simulink model "CF009A_GmOvrlStMgr"  (R2013b)
settings: Solver=FixedStepDiscrete  SolverMode=SingleTasking  StartTime=0.0  StopTime=1  FixedStep=0.002  RelTol=1e-3
values from neighbouring files (symbols this model uses):
  APASTACTV_CNT_U08 = DataDict.Constant    [CF009A_GmOvrlStMgr_DataDict.m]
  APASTCTRLAVL_CNT_U08 = DataDict.Constant    [CF009A_GmOvrlStMgr_DataDict.m]
  ARCHGLBPRM_2MILLISEC_SEC_F32 = DataDict.Constant    [CF009A_GmOvrlStMgr_DataDict.m]
  GmOvrlStMgrApaHwTqThd = DataDict.Calibration    [CF009A_GmOvrlStMgr_DataDict.m]
  GmOvrlStMgrApaHwTqTiThd = DataDict.Calibration    [CF009A_GmOvrlStMgr_DataDict.m]
  GmOvrlStMgrApaMfgEna = DataDict.Calibration    [CF009A_GmOvrlStMgr_DataDict.m]
  GmOvrlStMgrEscMfgEna = DataDict.Calibration    [CF009A_GmOvrlStMgr_DataDict.m]
  GmOvrlStMgrHaptcAmp = DataDict.Calibration    [CF009A_GmOvrlStMgr_DataDict.m]
  GmOvrlStMgrHaptcDurn = DataDict.Calibration    [CF009A_GmOvrlStMgr_DataDict.m]
  GmOvrlStMgrHaptcFrq = DataDict.Calibration    [CF009A_GmOvrlStMgr_DataDict.m]
  GmOvrlStMgrHaptcReactnTi = DataDict.Calibration    [CF009A_GmOvrlStMgr_DataDict.m]
  GmOvrlStMgrHaptcReqTiThd = DataDict.Calibration    [CF009A_GmOvrlStMgr_DataDict.m]
  GmOvrlStMgrHwAgTarLimr = DataDict.Calibration    [CF009A_GmOvrlStMgr_DataDict.m]
  GmOvrlStMgrLkaHwTqThd1 = DataDict.Calibration    [CF009A_GmOvrlStMgr_DataDict.m]
  GmOvrlStMgrLkaHwTqThd2 = DataDict.Calibration    [CF009A_GmOvrlStMgr_DataDict.m]
  GmOvrlStMgrLkaHwTqTiThd1 = DataDict.Calibration    [CF009A_GmOvrlStMgr_DataDict.m]
  GmOvrlStMgrLkaHwTqTiThd2 = DataDict.Calibration    [CF009A_GmOvrlStMgr_DataDict.m]
  GmOvrlStMgrLkaMfgEna = DataDict.Calibration    [CF009A_GmOvrlStMgr_DataDict.m]
  GmOvrlStMgrLoaMtgtnHaptcFbOffTi = DataDict.Calibration    [CF009A_GmOvrlStMgr_DataDict.m]
  GmOvrlStMgrLoaMtgtnHaptcFbOnTi = DataDict.Calibration    [CF009A_GmOvrlStMgr_DataDict.m]
  GmOvrlStMgrLoaMtgtnHaptcFbStrtOnTi = DataDict.Calibration    [CF009A_GmOvrlStMgr_DataDict.m]
  GmOvrlStMgrLoaMtgtnHaptcFbTqMax = DataDict.Calibration    [CF009A_GmOvrlStMgr_DataDict.m]
  GmOvrlStMgrLoaMtgtnHaptcFbTqMin = DataDict.Calibration    [CF009A_GmOvrlStMgr_DataDict.m]
  GmOvrlStMgrLoaMtgtnHaptcFbVehSpdMax = DataDict.Calibration    [CF009A_GmOvrlStMgr_DataDict.m]
  GmOvrlStMgrLoaMtgtnHaptcFbVehSpdMin = DataDict.Calibration    [CF009A_GmOvrlStMgr_DataDict.m]
  GmOvrlStMgrLoaMtgtnHaptcFrq = DataDict.Calibration    [CF009A_GmOvrlStMgr_DataDict.m]
  GmOvrlStMgrLoaMtgtnStrtHaptcAmp = DataDict.Calibration    [CF009A_GmOvrlStMgr_DataDict.m]
  GmOvrlStMgrLoaStIgnCntrThd = DataDict.Calibration    [CF009A_GmOvrlStMgr_DataDict.m]
  GmOvrlStMgrShiftLvrTiThd = DataDict.Calibration    [CF009A_GmOvrlStMgr_DataDict.m]
  GmOvrlStMgrStandStillThd = DataDict.Calibration    [CF009A_GmOvrlStMgr_DataDict.m]
  GmOvrlStMgrStandStillTiThd = DataDict.Calibration    [CF009A_GmOvrlStMgr_DataDict.m]
  HAPTCSTACTV_CNT_U08 = DataDict.Constant    [CF009A_GmOvrlStMgr_DataDict.m]
  HAPTCSTWAIT_CNT_U08 = DataDict.Constant    [CF009A_GmOvrlStMgr_DataDict.m]
  HWOSCNFRQMIN_HZ_F32 = DataDict.Constant    [CF009A_GmOvrlStMgr_DataDict.m]
  LKAFLTCNTRTHD_CNT_U08 = DataDict.Constant    [CF009A_GmOvrlStMgr_DataDict.m]
  LKAFLTTMRTHD_MILLISEC_U32 = DataDict.Constant    [CF009A_GmOvrlStMgr_DataDict.m]
  LKASTPRMNTFAILD_CNT_U08 = DataDict.Constant    [CF009A_GmOvrlStMgr_DataDict.m]
  LoaMtgtnThdExcdd = DataDict.NTC    [CF009A_GmOvrlStMgr_DataDict.m]
  MILLISECTO100MICROSECCNVN_CNT_U32 = DataDict.Constant    [CF009A_GmOvrlStMgr_DataDict.m]
  NODEBSTEP_CNT_U16 = DataDict.Constant    [CF009A_GmOvrlStMgr_DataDict.m]
undefined symbols (not defined in the file or in its folder): LoaSt1, NtcSts1, NVM_RequestResultType, SysSt1
libraries: simulink x13, Fil x6, NxtrNvM x4, NxtrLim x4, NxtrAbslt x3, NxtrSign x2, FixdToFloat x1, FloatToFixd x1, LnrIntrpn x1
(part 6 of 8)

== system CF009A_GmOvrlStMgr/GmOvrlStMgr/GmOvrlStMgrPer1/Timer for HwHaptcEna/If Action Subsystem/GetRefTmr100MicroSec32bit ==
  note: GetRefTmr100MicroSec32bit
  note: Wrap-to-zero
  note: counts
  note: microseconds
  note: seconds
  note: 1 count = 100 uSec
  CopyRight2 : Subsystem  Description=|  mask(Copyright Information){none=on}
      | Copyright info block.                                               
      |                                                                     
      | Place copyright information at the top of every subsystem in design.
      mask prompts: none "No parameters"
      mask help: Place copyright information at the top of every subsystem in design.
      mask Display:
      | NxtrConf = 'Nexteer Confidential';
      | 
      | sys = bdroot; %handle for the current model ("system")
      | first = get_param(sys,'Created');
      | if(isempty(first))
      |     first = datestr(now,'yyyy');
      | else
      |     first = first(end-3:end);  %year is last four digits
      | end
      | 
      | last = get_param(sys,'LastModifiedDate');
      | if isempty(last)
      |     last = datestr(now,'yyyy');
      | else
      |     last = last(end-3:end);
      | end
      | 
      | if strcmp(first,last)
      |     fprintf('%s -- Copyright %s Nexteer',NxtrConf,first)
      | else
      |     fprintf('%s -- %s%s- %s Nexteer',NxtrConf,char(169),first,last)
      | end
  Count per uSec : Constant  Value=0.01
  Data Store Read1 : DataStoreRead  DataStoreName=SimnTi
  Data Type Conversion1 : DataTypeConversion  OutDataTypeStr=uint32
  Divide1 : Product  Inputs=**
  Divide2 : Product  Inputs=*/
  Max Counts : Constant  Value=2^32-1
  Product1 : Product
  Product2 : Product
  Rounding : Rounding
  Subtract1 : Sum  Inputs=+-
  uSec per Sec : Constant  Value=1000000
  RefTmr : Outport
  wires:
  Data Type Conversion1/1 -> RefTmr/1
  uSec per Sec/1 -> Product1/2
  Count per uSec/1 -> Divide1/2
  Data Store Read1/1 -> Product1/1
  Product1/1 -> Divide1/1
  Divide1/1 -> Subtract1/1, Divide2/1
  Max Counts/1 -> Product2/2, Divide2/2
  Divide2/1 -> Rounding/1
  Rounding/1 -> Product2/1
  Subtract1/1 -> Data Type Conversion1/1
  Product2/1 -> Subtract1/2

== system CF009A_GmOvrlStMgr/GmOvrlStMgr/GmOvrlStMgrPer1/Timer for HwHaptcEna/If Action Subsystem1/CopyRight2 ==

== system CF009A_GmOvrlStMgr/GmOvrlStMgr/GmOvrlStMgrPer1/Timer for HwHaptcEna/If Action Subsystem2/CopyRight2 ==

== system CF009A_GmOvrlStMgr/GmOvrlStMgr/GmOvrlStMgrPer1/Timer for HwHaptcEna/If Action Subsystem2/GetTiSpan100MicroSec32bit1 ==
  note: GetTiSpan100MicroSec32bit
  note: Get current system time
  note: 1 count = 100 uSec
  note: Wrap-to-zero
  note: counts
  note: microseconds
  note: seconds
  note: Subtract original reference time
  RefTmr : Inport
  CopyRight2 : Subsystem  Description=|  mask(Copyright Information){none=on}
      | Copyright info block.                                               
      |                                                                     
      | Place copyright information at the top of every subsystem in design.
      mask prompts: none "No parameters"
      mask help: Place copyright information at the top of every subsystem in design.
      mask Display:
      | NxtrConf = 'Nexteer Confidential';
      | 
      | sys = bdroot; %handle for the current model ("system")
      | first = get_param(sys,'Created');
      | if(isempty(first))
      |     first = datestr(now,'yyyy');
      | else
      |     first = first(end-3:end);  %year is last four digits
      | end
      | 
      | last = get_param(sys,'LastModifiedDate');
      | if isempty(last)
      |     last = datestr(now,'yyyy');
      | else
      |     last = last(end-3:end);
      | end
      | 
      | if strcmp(first,last)
      |     fprintf('%s -- Copyright %s Nexteer',NxtrConf,first)
      | else
      |     fprintf('%s -- %s%s- %s Nexteer',NxtrConf,char(169),first,last)
      | end
  Count per uSec : Constant  Value=0.01
  Data Store Read1 : DataStoreRead  DataStoreName=SimnTi
  Data Type Conversion2 : DataTypeConversion  OutDataTypeStr=uint32
  Divide1 : Product  Inputs=**
  Divide2 : Product  Inputs=*/
  If : If  NumInputs=2  IfExpression=u1 >= u2
  Max Counts : Constant  Value=2^32-1
  Merge : Merge
  No wrapping : Subsystem  TreatAsAtomicUnit=on
  Product2 : Product
  Product3 : Product
  Rounding : Rounding
  Subtract3 : Sum  Inputs=+-
  Wrapping : Subsystem  TreatAsAtomicUnit=on
  uSec per Sec : Constant  Value=1000000
  TiSpan : Outport
  wires:
  Data Type Conversion2/1 -> Wrapping/1(new), No wrapping/1(new), If/1
  RefTmr/1 -> Wrapping/2(ref), No wrapping/2(ref), If/2
  Merge/1 -> TiSpan/1
  uSec per Sec/1 -> Product2/2
  Count per uSec/1 -> Divide1/2
  Data Store Read1/1 -> Product2/1
  Product2/1 -> Divide1/1
  Divide1/1 -> Subtract3/1, Divide2/1
  Max Counts/1 -> Product3/2, Divide2/2
  Divide2/1 -> Rounding/1
  Rounding/1 -> Product3/1
  Subtract3/1 -> Data Type Conversion2/1
  Product3/1 -> Subtract3/2
  If/1 -> No wrapping/Action
  If/2 -> Wrapping/Action
  No wrapping/1(Out1) -> Merge/1
  Wrapping/1(Out1) -> Merge/2

== system CF009A_GmOvrlStMgr/GmOvrlStMgr/GmOvrlStMgrPer1/Timer for ShiftLvrRvs/If Action Subsystem/CopyRight2 ==

== system CF009A_GmOvrlStMgr/GmOvrlStMgr/GmOvrlStMgrPer1/Timer for ShiftLvrRvs/If Action Subsystem/GetRefTmr100MicroSec32bit ==
  note: GetRefTmr100MicroSec32bit
  note: Wrap-to-zero
  note: counts
  note: microseconds
  note: seconds
  note: 1 count = 100 uSec
  CopyRight2 : Subsystem  Description=|  mask(Copyright Information){none=on}
      | Copyright info block.                                               
      |                                                                     
      | Place copyright information at the top of every subsystem in design.
      mask prompts: none "No parameters"
      mask help: Place copyright information at the top of every subsystem in design.
      mask Display:
      | NxtrConf = 'Nexteer Confidential';
      | 
      | sys = bdroot; %handle for the current model ("system")
      | first = get_param(sys,'Created');
      | if(isempty(first))
      |     first = datestr(now,'yyyy');
      | else
      |     first = first(end-3:end);  %year is last four digits
      | end
      | 
      | last = get_param(sys,'LastModifiedDate');
      | if isempty(last)
      |     last = datestr(now,'yyyy');
      | else
      |     last = last(end-3:end);
      | end
      | 
      | if strcmp(first,last)
      |     fprintf('%s -- Copyright %s Nexteer',NxtrConf,first)
      | else
      |     fprintf('%s -- %s%s- %s Nexteer',NxtrConf,char(169),first,last)
      | end
  Count per uSec : Constant  Value=0.01
  Data Store Read1 : DataStoreRead  DataStoreName=SimnTi
  Data Type Conversion1 : DataTypeConversion  OutDataTypeStr=uint32
  Divide1 : Product  Inputs=**
  Divide2 : Product  Inputs=*/
  Max Counts : Constant  Value=2^32-1
  Product1 : Product
  Product2 : Product
  Rounding : Rounding
  Subtract1 : Sum  Inputs=+-
  uSec per Sec : Constant  Value=1000000
  RefTmr : Outport
  wires:
  Data Type Conversion1/1 -> RefTmr/1
  uSec per Sec/1 -> Product1/2
  Count per uSec/1 -> Divide1/2
  Data Store Read1/1 -> Product1/1
  Product1/1 -> Divide1/1
  Divide1/1 -> Subtract1/1, Divide2/1
  Max Counts/1 -> Product2/2, Divide2/2
  Divide2/1 -> Rounding/1
  Rounding/1 -> Product2/1
  Subtract1/1 -> Data Type Conversion1/1
  Product2/1 -> Subtract1/2

== system CF009A_GmOvrlStMgr/GmOvrlStMgr/GmOvrlStMgrPer1/Timer for ShiftLvrRvs/If Action Subsystem1/CopyRight2 ==

== system CF009A_GmOvrlStMgr/GmOvrlStMgr/GmOvrlStMgrPer1/Timer for ShiftLvrRvs/If Action Subsystem2/CopyRight2 ==

== system CF009A_GmOvrlStMgr/GmOvrlStMgr/GmOvrlStMgrPer1/Timer for ShiftLvrRvs/If Action Subsystem2/GetTiSpan100MicroSec32bit1 ==
  note: GetTiSpan100MicroSec32bit
  note: Get current system time
  note: 1 count = 100 uSec
  note: Wrap-to-zero
  note: counts
  note: microseconds
  note: seconds
  note: Subtract original reference time
  RefTmr : Inport
  CopyRight2 : Subsystem  Description=|  mask(Copyright Information){none=on}
      | Copyright info block.                                               
      |                                                                     
      | Place copyright information at the top of every subsystem in design.
      mask prompts: none "No parameters"
      mask help: Place copyright information at the top of every subsystem in design.
      mask Display:
      | NxtrConf = 'Nexteer Confidential';
      | 
      | sys = bdroot; %handle for the current model ("system")
      | first = get_param(sys,'Created');
      | if(isempty(first))
      |     first = datestr(now,'yyyy');
      | else
      |     first = first(end-3:end);  %year is last four digits
      | end
      | 
      | last = get_param(sys,'LastModifiedDate');
      | if isempty(last)
      |     last = datestr(now,'yyyy');
      | else
      |     last = last(end-3:end);
      | end
      | 
      | if strcmp(first,last)
      |     fprintf('%s -- Copyright %s Nexteer',NxtrConf,first)
      | else
      |     fprintf('%s -- %s%s- %s Nexteer',NxtrConf,char(169),first,last)
      | end
  Count per uSec : Constant  Value=0.01
  Data Store Read1 : DataStoreRead  DataStoreName=SimnTi
  Data Type Conversion2 : DataTypeConversion  OutDataTypeStr=uint32
  Divide1 : Product  Inputs=**
  Divide2 : Product  Inputs=*/
  If : If  NumInputs=2  IfExpression=u1 >= u2
  Max Counts : Constant  Value=2^32-1
  Merge : Merge
  No wrapping : Subsystem  TreatAsAtomicUnit=on
  Product2 : Product
  Product3 : Product
  Rounding : Rounding
  Subtract3 : Sum  Inputs=+-
  Wrapping : Subsystem  TreatAsAtomicUnit=on
  uSec per Sec : Constant  Value=1000000
  TiSpan : Outport
  wires:
  Data Type Conversion2/1 -> Wrapping/1(new), No wrapping/1(new), If/1
  RefTmr/1 -> Wrapping/2(ref), No wrapping/2(ref), If/2
  Merge/1 -> TiSpan/1
  uSec per Sec/1 -> Product2/2
  Count per uSec/1 -> Divide1/2
  Data Store Read1/1 -> Product2/1
  Product2/1 -> Divide1/1
  Divide1/1 -> Subtract3/1, Divide2/1
  Max Counts/1 -> Product3/2, Divide2/2
  Divide2/1 -> Rounding/1
  Rounding/1 -> Product3/1
  Subtract3/1 -> Data Type Conversion2/1
  Product3/1 -> Subtract3/2
  If/1 -> No wrapping/Action
  If/2 -> Wrapping/Action
  No wrapping/1(Out1) -> Merge/1
  Wrapping/1(Out1) -> Merge/2

== system CF009A_GmOvrlStMgr/GmOvrlStMgr/GmOvrlStMgrPer1/Timer for VehStandStill/If Action Subsystem/CopyRight2 ==

== system CF009A_GmOvrlStMgr/GmOvrlStMgr/GmOvrlStMgrPer1/Timer for VehStandStill/If Action Subsystem/GetRefTmr100MicroSec32bit ==
  note: GetRefTmr100MicroSec32bit
  note: Wrap-to-zero
  note: counts
  note: microseconds
  note: seconds
  note: 1 count = 100 uSec
  CopyRight2 : Subsystem  Description=|  mask(Copyright Information){none=on}
      | Copyright info block.                                               
      |                                                                     
      | Place copyright information at the top of every subsystem in design.
      mask prompts: none "No parameters"
      mask help: Place copyright information at the top of every subsystem in design.
      mask Display:
      | NxtrConf = 'Nexteer Confidential';
      | 
      | sys = bdroot; %handle for the current model ("system")
      | first = get_param(sys,'Created');
      | if(isempty(first))
      |     first = datestr(now,'yyyy');
      | else
      |     first = first(end-3:end);  %year is last four digits
      | end
      | 
      | last = get_param(sys,'LastModifiedDate');
      | if isempty(last)
      |     last = datestr(now,'yyyy');
      | else
      |     last = last(end-3:end);
      | end
      | 
      | if strcmp(first,last)
      |     fprintf('%s -- Copyright %s Nexteer',NxtrConf,first)
      | else
      |     fprintf('%s -- %s%s- %s Nexteer',NxtrConf,char(169),first,last)
      | end
  Count per uSec : Constant  Value=0.01
  Data Store Read1 : DataStoreRead  DataStoreName=SimnTi
  Data Type Conversion1 : DataTypeConversion  OutDataTypeStr=uint32
  Divide1 : Product  Inputs=**
  Divide2 : Product  Inputs=*/
  Max Counts : Constant  Value=2^32-1
  Product1 : Product
  Product2 : Product
  Rounding : Rounding
  Subtract1 : Sum  Inputs=+-
  uSec per Sec : Constant  Value=1000000
  RefTmr : Outport
  wires:
  Data Type Conversion1/1 -> RefTmr/1
  uSec per Sec/1 -> Product1/2
  Count per uSec/1 -> Divide1/2
  Data Store Read1/1 -> Product1/1
  Product1/1 -> Divide1/1
  Divide1/1 -> Subtract1/1, Divide2/1
  Max Counts/1 -> Product2/2, Divide2/2
  Divide2/1 -> Rounding/1
  Rounding/1 -> Product2/1
  Subtract1/1 -> Data Type Conversion1/1
  Product2/1 -> Subtract1/2

== system CF009A_GmOvrlStMgr/GmOvrlStMgr/GmOvrlStMgrPer1/Timer for VehStandStill/If Action Subsystem1/CopyRight2 ==

== system CF009A_GmOvrlStMgr/GmOvrlStMgr/GmOvrlStMgrPer1/Timer for VehStandStill/If Action Subsystem2/CopyRight2 ==

== system CF009A_GmOvrlStMgr/GmOvrlStMgr/GmOvrlStMgrPer1/Timer for VehStandStill/If Action Subsystem2/GetTiSpan100MicroSec32bit1 ==
  note: GetTiSpan100MicroSec32bit
  note: Get current system time
  note: 1 count = 100 uSec
  note: Wrap-to-zero
  note: counts
  note: microseconds
  note: seconds
  note: Subtract original reference time
  RefTmr : Inport
  CopyRight2 : Subsystem  Description=|  mask(Copyright Information){none=on}
      | Copyright info block.                                               
      |                                                                     
      | Place copyright information at the top of every subsystem in design.
      mask prompts: none "No parameters"
      mask help: Place copyright information at the top of every subsystem in design.
      mask Display:
      | NxtrConf = 'Nexteer Confidential';
      | 
      | sys = bdroot; %handle for the current model ("system")
      | first = get_param(sys,'Created');
      | if(isempty(first))
      |     first = datestr(now,'yyyy');
      | else
      |     first = first(end-3:end);  %year is last four digits
      | end
      | 
      | last = get_param(sys,'LastModifiedDate');
      | if isempty(last)
      |     last = datestr(now,'yyyy');
      | else
      |     last = last(end-3:end);
      | end
      | 
      | if strcmp(first,last)
      |     fprintf('%s -- Copyright %s Nexteer',NxtrConf,first)
      | else
      |     fprintf('%s -- %s%s- %s Nexteer',NxtrConf,char(169),first,last)
      | end
  Count per uSec : Constant  Value=0.01
  Data Store Read1 : DataStoreRead  DataStoreName=SimnTi
  Data Type Conversion2 : DataTypeConversion  OutDataTypeStr=uint32
  Divide1 : Product  Inputs=**
  Divide2 : Product  Inputs=*/
  If : If  NumInputs=2  IfExpression=u1 >= u2
  Max Counts : Constant  Value=2^32-1
  Merge : Merge
  No wrapping : Subsystem  TreatAsAtomicUnit=on
  Product2 : Product
  Product3 : Product
  Rounding : Rounding
  Subtract3 : Sum  Inputs=+-
  Wrapping : Subsystem  TreatAsAtomicUnit=on
  uSec per Sec : Constant  Value=1000000
  TiSpan : Outport
  wires:
  Data Type Conversion2/1 -> Wrapping/1(new), No wrapping/1(new), If/1
  RefTmr/1 -> Wrapping/2(ref), No wrapping/2(ref), If/2
  Merge/1 -> TiSpan/1
  uSec per Sec/1 -> Product2/2
  Count per uSec/1 -> Divide1/2
  Data Store Read1/1 -> Product2/1
  Product2/1 -> Divide1/1
  Divide1/1 -> Subtract3/1, Divide2/1
  Max Counts/1 -> Product3/2, Divide2/2
  Divide2/1 -> Rounding/1
  Rounding/1 -> Product3/1
  Subtract3/1 -> Data Type Conversion2/1
  Product3/1 -> Subtract3/2
  If/1 -> No wrapping/Action
  If/2 -> Wrapping/Action
  No wrapping/1(Out1) -> Merge/1
  Wrapping/1(Out1) -> Merge/2

== system CF009A_GmOvrlStMgr/GmOvrlStMgr/GmOvrlStMgrPer1/TransHaptcsWaitToAPAStActvFlg/ElpseTi/CopyRight2 ==

== system CF009A_GmOvrlStMgr/GmOvrlStMgr/GmOvrlStMgrPer1/TransHaptcsWaitToAPAStActvFlg/ElpseTi/GetTiSpan100MicroSec32bit ==
  note: Created Aug 18, 2015
      | Modified Oct 21, 2015
      | Modified Oct 30, 2015
      | Kevin Derry
  note: GetTiSpan100MicroSec32bit
  note: Get current system time
  note: 1 count = 100 uSec
  note: Wrap-to-zero
  note: counts
  note: microseconds
  note: seconds
  note: Subtract original reference time
  RefTmr : Inport
  CopyRight2 : Subsystem  Description=|  mask(Copyright Information){none=on}
      | Copyright info block.                                               
      |                                                                     
      | Place copyright information at the top of every subsystem in design.
      mask prompts: none "No parameters"
      mask help: Place copyright information at the top of every subsystem in design.
      mask Display:
      | NxtrConf = 'Nexteer Confidential';
      | 
      | sys = bdroot; %handle for the current model ("system")
      | first = get_param(sys,'Created');
      | if(isempty(first))
      |     first = datestr(now,'yyyy');
      | else
      |     first = first(end-3:end);  %year is last four digits
      | end
      | 
      | last = get_param(sys,'LastModifiedDate');
      | if isempty(last)
      |     last = datestr(now,'yyyy');
      | else
      |     last = last(end-3:end);
      | end
      | 
      | if strcmp(first,last)
      |     fprintf('%s -- Copyright %s Nexteer',NxtrConf,first)
      | else
      |     fprintf('%s -- %s%s- %s Nexteer',NxtrConf,char(169),first,last)
      | end
  Count per uSec : Constant  Value=0.01
  Data Store Read1 : DataStoreRead  DataStoreName=SimnTi
  Data Type Conversion2 : DataTypeConversion  OutDataTypeStr=uint32
  Divide1 : Product  Inputs=**
  Divide2 : Product  Inputs=*/
  If : If  NumInputs=2  IfExpression=u1 >= u2
  Max Counts : Constant  Value=2^32-1
  Merge : Merge
  No wrapping : Subsystem  TreatAsAtomicUnit=on
  Product2 : Product
  Product3 : Product
  Rounding : Rounding
  Subtract3 : Sum  Inputs=+-
  Wrapping : Subsystem  TreatAsAtomicUnit=on
  uSec per Sec : Constant  Value=1000000
  TiSpan : Outport
  wires:
  Data Type Conversion2/1 -> Wrapping/1(new), No wrapping/1(new), If/1
  RefTmr/1 -> Wrapping/2(ref), No wrapping/2(ref), If/2
  Merge/1 -> TiSpan/1
  uSec per Sec/1 -> Product2/2
  Count per uSec/1 -> Divide1/2
  Data Store Read1/1 -> Product2/1
  Product2/1 -> Divide1/1
  Divide1/1 -> Subtract3/1, Divide2/1
  Max Counts/1 -> Product3/2, Divide2/2
  Divide2/1 -> Rounding/1
  Rounding/1 -> Product3/1
  Subtract3/1 -> Data Type Conversion2/1
  Product3/1 -> Subtract3/2
  If/1 -> No wrapping/Action
  If/2 -> Wrapping/Action
  No wrapping/1(Out1) -> Merge/1
  Wrapping/1(Out1) -> Merge/2

== system CF009A_GmOvrlStMgr/GmOvrlStMgr/GmOvrlStMgrPer1/TransHaptcsWaitToAPAStActvFlg/ElpseTi/Set False Subsystem ==
  Action Port : ActionPort  ActionType=else
  Constant1 : Constant  RequirementInfo={} %GIDa_654f473a_f2a5_43e8_8504_41bd23fb1d71  Value=false  OutDataTypeStr=boolean
      settings: AttributesFormatString=%<OutDataTypeStr>
  CopyRight2 : Subsystem  Description=|  mask(Copyright Information){none=on}
      | Copyright info block.                                               
      |                                                                     
      | Place copyright information at the top of every subsystem in design.
      mask prompts: none "No parameters"
      mask help: Place copyright information at the top of every subsystem in design.
      mask Display:
      | NxtrConf = 'Nexteer Confidential';
      | 
      | sys = bdroot; %handle for the current model ("system")
      | first = get_param(sys,'Created');
      | first = first(end-3:end);  %year is last four digits
      | 
      | last = get_param(sys,'LastModifiedDate');
      | if isempty(last)
      |     last = datestr(now,'yyyy');
      | else
      |     last = last(end-3:end);
      | end
      | 
      | if strcmp(first,last)
      |     fprintf('%s -- Copyright %s Nexteer',NxtrConf,first)
      | else
      |     fprintf('%s -- %s%s- %s Nexteer',NxtrConf,char(169),first,last)
      | end
  Out1 : Outport
  wires:
  Constant1/1 -> Out1/1

== system CF009A_GmOvrlStMgr/GmOvrlStMgr/GmOvrlStMgrPer1/TransHaptcsWaitToAPAStActvFlg/ElpseTi/Set True Subsystem ==
  Action Port : ActionPort  ActionType=then
  Constant13 : Constant  RequirementInfo={} %GIDa_d24888ab_9be7_4cc6_a531_95638502a8a2  Value=true  OutDataTypeStr=boolean
      settings: AttributesFormatString=%<OutDataTypeStr>
  CopyRight2 : Subsystem  Description=|  mask(Copyright Information){none=on}
      | Copyright info block.                                               
      |                                                                     
      | Place copyright information at the top of every subsystem in design.
      mask prompts: none "No parameters"
      mask help: Place copyright information at the top of every subsystem in design.
      mask Display:
      | NxtrConf = 'Nexteer Confidential';
      | 
      | sys = bdroot; %handle for the current model ("system")
      | first = get_param(sys,'Created');
      | first = first(end-3:end);  %year is last four digits
      | 
      | last = get_param(sys,'LastModifiedDate');
      | if isempty(last)
      |     last = datestr(now,'yyyy');
      | else
      |     last = last(end-3:end);
      | end
      | 
      | if strcmp(first,last)
      |     fprintf('%s -- Copyright %s Nexteer',NxtrConf,first)
      | else
      |     fprintf('%s -- %s%s- %s Nexteer',NxtrConf,char(169),first,last)
      | end
  Out1 : Outport
  wires:
  Constant13/1 -> Out1/1

== system CF009A_GmOvrlStMgr/GmOvrlStMgr/GmOvrlStMgrPer1/TransHaptcsWaitToAPAStActvFlg/RefTi/CopyRight2 ==

== system CF009A_GmOvrlStMgr/GmOvrlStMgr/GmOvrlStMgrPer1/TransHaptcsWaitToAPAStActvFlg/RefTi/GetRefTmr100MicroSec32bit ==
  note: Created Aug 18, 2015
      | Modified Oct 21, 2015
      | Modified Oct 30, 2015
      | Kevin Derry
  note: GetRefTmr100MicroSec32bit
  note: Wrap-to-zero
  note: counts
  note: microseconds
  note: seconds
  note: 1 count = 100 uSec
  CopyRight2 : Subsystem  Description=|  mask(Copyright Information){none=on}
      | Copyright info block.                                               
      |                                                                     
      | Place copyright information at the top of every subsystem in design.
      mask prompts: none "No parameters"
      mask help: Place copyright information at the top of every subsystem in design.
      mask Display:
      | NxtrConf = 'Nexteer Confidential';
      | 
      | sys = bdroot; %handle for the current model ("system")
      | first = get_param(sys,'Created');
      | if(isempty(first))
      |     first = datestr(now,'yyyy');
      | else
      |     first = first(end-3:end);  %year is last four digits
      | end
      | 
      | last = get_param(sys,'LastModifiedDate');
      | if isempty(last)
      |     last = datestr(now,'yyyy');
      | else
      |     last = last(end-3:end);
      | end
      | 
      | if strcmp(first,last)
      |     fprintf('%s -- Copyright %s Nexteer',NxtrConf,first)
      | else
      |     fprintf('%s -- %s%s- %s Nexteer',NxtrConf,char(169),first,last)
      | end
  Count per uSec : Constant  Value=0.01
  Data Store Read1 : DataStoreRead  DataStoreName=SimnTi
  Data Type Conversion1 : DataTypeConversion  OutDataTypeStr=uint32
  Divide1 : Product  Inputs=**
  Divide2 : Product  Inputs=*/
  Max Counts : Constant  Value=2^32-1
  Product1 : Product
  Product2 : Product
  Rounding : Rounding
  Subtract1 : Sum  Inputs=+-
  uSec per Sec : Constant  Value=1000000
  RefTmr : Outport
  wires:
  Data Store Read1/1 -> Product1/1
  Data Type Conversion1/1 -> RefTmr/1
  uSec per Sec/1 -> Product1/2
  Count per uSec/1 -> Divide1/2
  Product1/1 -> Divide1/1
  Divide1/1 -> Subtract1/1, Divide2/1
  Max Counts/1 -> Product2/2, Divide2/2
  Divide2/1 -> Rounding/1
  Rounding/1 -> Product2/1
  Subtract1/1 -> Data Type Conversion1/1
  Product2/1 -> Subtract1/2

== system CF009A_GmOvrlStMgr/GmOvrlStMgr/GmOvrlStMgrPer1/ApaIntv/Timer for ApaIntv/If Action Subsystem/CopyRight2 ==

== system CF009A_GmOvrlStMgr/GmOvrlStMgr/GmOvrlStMgrPer1/ApaIntv/Timer for ApaIntv/If Action Subsystem/GetRefTmr100MicroSec32bit ==
  note: GetRefTmr100MicroSec32bit
  note: Wrap-to-zero
  note: counts
  note: microseconds
  note: seconds
  note: 1 count = 100 uSec
  CopyRight2 : Subsystem  Description=|  mask(Copyright Information){none=on}
      | Copyright info block.                                               
      |                                                                     
      | Place copyright information at the top of every subsystem in design.
      mask prompts: none "No parameters"
      mask help: Place copyright information at the top of every subsystem in design.
      mask Display:
      | NxtrConf = 'Nexteer Confidential';
      | 
      | sys = bdroot; %handle for the current model ("system")
      | first = get_param(sys,'Created');
      | if(isempty(first))
      |     first = datestr(now,'yyyy');
      | else
      |     first = first(end-3:end);  %year is last four digits
      | end
      | 
      | last = get_param(sys,'LastModifiedDate');
      | if isempty(last)
      |     last = datestr(now,'yyyy');
      | else
      |     last = last(end-3:end);
      | end
      | 
      | if strcmp(first,last)
      |     fprintf('%s -- Copyright %s Nexteer',NxtrConf,first)
      | else
      |     fprintf('%s -- %s%s- %s Nexteer',NxtrConf,char(169),first,last)
      | end
  Count per uSec : Constant  Value=0.01
  Data Store Read1 : DataStoreRead  DataStoreName=SimnTi
  Data Type Conversion1 : DataTypeConversion  OutDataTypeStr=uint32
  Divide1 : Product  Inputs=**
  Divide2 : Product  Inputs=*/
  Max Counts : Constant  Value=2^32-1
  Product1 : Product
  Product2 : Product
  Rounding : Rounding
  Subtract1 : Sum  Inputs=+-
  uSec per Sec : Constant  Value=1000000
  RefTmr : Outport
  wires:
  Data Type Conversion1/1 -> RefTmr/1
  uSec per Sec/1 -> Product1/2
  Count per uSec/1 -> Divide1/2
  Data Store Read1/1 -> Product1/1
  Product1/1 -> Divide1/1
  Divide1/1 -> Subtract1/1, Divide2/1
  Max Counts/1 -> Product2/2, Divide2/2
  Divide2/1 -> Rounding/1
  Rounding/1 -> Product2/1
  Subtract1/1 -> Data Type Conversion1/1
  Product2/1 -> Subtract1/2

== system CF009A_GmOvrlStMgr/GmOvrlStMgr/GmOvrlStMgrPer1/ApaIntv/Timer for ApaIntv/If Action Subsystem1/CopyRight2 ==

== system CF009A_GmOvrlStMgr/GmOvrlStMgr/GmOvrlStMgrPer1/ApaIntv/Timer for ApaIntv/If Action Subsystem2/CopyRight2 ==

== system CF009A_GmOvrlStMgr/GmOvrlStMgr/GmOvrlStMgrPer1/ApaIntv/Timer for ApaIntv/If Action Subsystem2/GetTiSpan100MicroSec32bit1 ==
  note: GetTiSpan100MicroSec32bit
  note: Get current system time
  note: 1 count = 100 uSec
  note: Wrap-to-zero
  note: counts
  note: microseconds
  note: seconds
  note: Subtract original reference time
  RefTmr : Inport
  CopyRight2 : Subsystem  Description=|  mask(Copyright Information){none=on}
      | Copyright info block.                                               
      |                                                                     
      | Place copyright information at the top of every subsystem in design.
      mask prompts: none "No parameters"
      mask help: Place copyright information at the top of every subsystem in design.
      mask Display:
      | NxtrConf = 'Nexteer Confidential';
      | 
      | sys = bdroot; %handle for the current model ("system")
      | first = get_param(sys,'Created');
      | if(isempty(first))
      |     first = datestr(now,'yyyy');
      | else
      |     first = first(end-3:end);  %year is last four digits
      | end
      | 
      | last = get_param(sys,'LastModifiedDate');
      | if isempty(last)
      |     last = datestr(now,'yyyy');
      | else
      |     last = last(end-3:end);
      | end
      | 
      | if strcmp(first,last)
      |     fprintf('%s -- Copyright %s Nexteer',NxtrConf,first)
      | else
      |     fprintf('%s -- %s%s- %s Nexteer',NxtrConf,char(169),first,last)
      | end
  Count per uSec : Constant  Value=0.01
  Data Store Read1 : DataStoreRead  DataStoreName=SimnTi
  Data Type Conversion2 : DataTypeConversion  OutDataTypeStr=uint32
  Divide1 : Product  Inputs=**
  Divide2 : Product  Inputs=*/
  If : If  NumInputs=2  IfExpression=u1 >= u2
  Max Counts : Constant  Value=2^32-1
  Merge : Merge
  No wrapping : Subsystem  TreatAsAtomicUnit=on
  Product2 : Product
  Product3 : Product
  Rounding : Rounding
  Subtract3 : Sum  Inputs=+-
  Wrapping : Subsystem  TreatAsAtomicUnit=on
  uSec per Sec : Constant  Value=1000000
  TiSpan : Outport
  wires:
  Data Type Conversion2/1 -> Wrapping/1(new), No wrapping/1(new), If/1
  RefTmr/1 -> Wrapping/2(ref), No wrapping/2(ref), If/2
  Merge/1 -> TiSpan/1
  uSec per Sec/1 -> Product2/2
  Count per uSec/1 -> Divide1/2
  Data Store Read1/1 -> Product2/1
  Product2/1 -> Divide1/1
  Divide1/1 -> Subtract3/1, Divide2/1
  Max Counts/1 -> Product3/2, Divide2/2
  Divide2/1 -> Rounding/1
  Rounding/1 -> Product3/1
  Subtract3/1 -> Data Type Conversion2/1
  Product3/1 -> Subtract3/2
  If/1 -> No wrapping/Action
  If/2 -> Wrapping/Action
  No wrapping/1(Out1) -> Merge/1
  Wrapping/1(Out1) -> Merge/2

== system CF009A_GmOvrlStMgr/GmOvrlStMgr/GmOvrlStMgrPer1/HaptcStTransActvToWaitFlg/ElpseTi/GetTiSpan100MicroSec32bit/CopyRight2 ==

== system CF009A_GmOvrlStMgr/GmOvrlStMgr/GmOvrlStMgrPer1/HaptcStTransActvToWaitFlg/ElpseTi/GetTiSpan100MicroSec32bit/No wrapping ==
  new : Inport
  ref : Inport  Port=2
  Action Port : ActionPort  ActionType=then
  CopyRight2 : Subsystem  Description=|  mask(Copyright Information){none=on}
      | Copyright info block.                                               
      |                                                                     
      | Place copyright information at the top of every subsystem in design.
      mask prompts: none "No parameters"
      mask help: Place copyright information at the top of every subsystem in design.
      mask Display:
      | NxtrConf = 'Nexteer Confidential';
      | 
      | sys = bdroot; %handle for the current model ("system")
      | first = get_param(sys,'Created');
      | if(isempty(first))
      |     first = datestr(now,'yyyy');
      | else
      |     first = first(end-3:end);  %year is last four digits
      | end
      | 
      | last = get_param(sys,'LastModifiedDate');
      | if isempty(last)
      |     last = datestr(now,'yyyy');
      | else
      |     last = last(end-3:end);
      | end
      | 
      | if strcmp(first,last)
      |     fprintf('%s -- Copyright %s Nexteer',NxtrConf,first)
      | else
      |     fprintf('%s -- %s%s- %s Nexteer',NxtrConf,char(169),first,last)
      | end
  Subtract1 : Sum  Inputs=+-
  Out1 : Outport
  wires:
  ref/1 -> Subtract1/2
  new/1 -> Subtract1/1
  Subtract1/1 -> Out1/1

== system CF009A_GmOvrlStMgr/GmOvrlStMgr/GmOvrlStMgrPer1/HaptcStTransActvToWaitFlg/ElpseTi/GetTiSpan100MicroSec32bit/Wrapping ==
  new : Inport
  ref : Inport  Port=2
  Action Port : ActionPort  ActionType=else
  CopyRight2 : Subsystem  Description=|  mask(Copyright Information){none=on}
      | Copyright info block.                                               
      |                                                                     
      | Place copyright information at the top of every subsystem in design.
      mask prompts: none "No parameters"
      mask help: Place copyright information at the top of every subsystem in design.
      mask Display:
      | NxtrConf = 'Nexteer Confidential';
      | 
      | sys = bdroot; %handle for the current model ("system")
      | first = get_param(sys,'Created');
      | if(isempty(first))
      |     first = datestr(now,'yyyy');
      | else
      |     first = first(end-3:end);  %year is last four digits
      | end
      | 
      | last = get_param(sys,'LastModifiedDate');
      | if isempty(last)
      |     last = datestr(now,'yyyy');
      | else
      |     last = last(end-3:end);
      | end
      | 
      | if strcmp(first,last)
      |     fprintf('%s -- Copyright %s Nexteer',NxtrConf,first)
      | else
      |     fprintf('%s -- %s%s- %s Nexteer',NxtrConf,char(169),first,last)
      | end
  Max Counts : Constant  Value=2^32-1  OutDataTypeStr=uint32
  Subtract1 : Sum  Inputs=+-+
  Out1 : Outport
  wires:
  new/1 -> Subtract1/3
  ref/1 -> Subtract1/2
  Max Counts/1 -> Subtract1/1
  Subtract1/1 -> Out1/1

== system CF009A_GmOvrlStMgr/GmOvrlStMgr/GmOvrlStMgrPer1/HaptcStTransActvToWaitFlg/ElpseTi/Set False Subsystem/CopyRight2 ==

== system CF009A_GmOvrlStMgr/GmOvrlStMgr/GmOvrlStMgrPer1/HaptcStTransActvToWaitFlg/ElpseTi/Set True Subsystem/CopyRight2 ==

== system CF009A_GmOvrlStMgr/GmOvrlStMgr/GmOvrlStMgrPer1/HaptcStTransActvToWaitFlg/RefTi/GetRefTmr100MicroSec32bit/CopyRight2 ==

== system CF009A_GmOvrlStMgr/GmOvrlStMgr/GmOvrlStMgrPer1/HwAgServo/If Action Subsystem/ApaStatusActive/CopyRight2 ==

== system CF009A_GmOvrlStMgr/GmOvrlStMgr/GmOvrlStMgrPer1/HwAgServo/If Action Subsystem/ApaStatusNotActive/CopyRight2 ==

== system CF009A_GmOvrlStMgr/GmOvrlStMgr/GmOvrlStMgrPer1/HwAgServo/If Action Subsystem1/ApaStatusActive/CopyRight2 ==

== system CF009A_GmOvrlStMgr/GmOvrlStMgr/GmOvrlStMgrPer1/HwAgServo/If Action Subsystem1/ApaStatusNotActive/CopyRight2 ==

== system CF009A_GmOvrlStMgr/GmOvrlStMgr/GmOvrlStMgrPer1/LKAIntv/HwTqLkaTqSignEqu/GetRefTmr100MicroSec32bit/CopyRight2 ==

== system CF009A_GmOvrlStMgr/GmOvrlStMgr/GmOvrlStMgrPer1/LKAIntv/HwTqLkaTqSignEqu/GetRefTmr100MicroSec32bit_1/CopyRight2 ==

== system CF009A_GmOvrlStMgr/GmOvrlStMgr/GmOvrlStMgrPer1/LKAIntv/HwTqLkaTqSignNotEqu/ChkTmr1/CopyRight2 ==

== system CF009A_GmOvrlStMgr/GmOvrlStMgr/GmOvrlStMgrPer1/LKAIntv/HwTqLkaTqSignNotEqu/ChkTmr1/GetRefTmr100MicroSec32bit ==
  note: 1 count = 100 uSec
  note: seconds
  note: microseconds
  note: counts
  note: Wrap-to-zero
  note: GetRefTmr100MicroSec32bit
  note: Created Aug 18, 2015
      | Modified Oct 21, 2015
      | Modified Oct 30, 2015
      | Kevin Derry
  CopyRight2 : Subsystem  Description=|  mask(Copyright Information){none=on}
      | Copyright info block.                                               
      |                                                                     
      | Place copyright information at the top of every subsystem in design.
      mask prompts: none "No parameters"
      mask help: Place copyright information at the top of every subsystem in design.
      mask Display:
      | NxtrConf = 'Nexteer Confidential';
      | 
      | sys = bdroot; %handle for the current model ("system")
      | first = get_param(sys,'Created');
      | if(isempty(first))
      |     first = datestr(now,'yyyy');
      | else
      |     first = first(end-3:end);  %year is last four digits
      | end
      | 
      | last = get_param(sys,'LastModifiedDate');
      | if isempty(last)
      |     last = datestr(now,'yyyy');
      | else
      |     last = last(end-3:end);
      | end
      | 
      | if strcmp(first,last)
      |     fprintf('%s -- Copyright %s Nexteer',NxtrConf,first)
      | else
      |     fprintf('%s -- %s%s- %s Nexteer',NxtrConf,char(169),first,last)
      | end
  Count per uSec : Constant  Value=0.01
  Data Store Read1 : DataStoreRead  DataStoreName=SimnTi
  Data Type Conversion1 : DataTypeConversion  OutDataTypeStr=uint32
  Divide1 : Product  Inputs=**
  Divide2 : Product  Inputs=*/
  Max Counts : Constant  Value=2^32-1
  Product1 : Product
  Product2 : Product
  Rounding : Rounding
  Subtract1 : Sum  Inputs=+-
  uSec per Sec : Constant  Value=1000000
  RefTmr : Outport
  wires:
  Product2/1 -> Subtract1/2
  Subtract1/1 -> Data Type Conversion1/1
  Rounding/1 -> Product2/1
  Divide2/1 -> Rounding/1
  Max Counts/1 -> Divide2/2, Product2/2
  Divide1/1 -> Divide2/1, Subtract1/1
  Product1/1 -> Divide1/1
  Count per uSec/1 -> Divide1/2
  uSec per Sec/1 -> Product1/2
  Data Type Conversion1/1 -> RefTmr/1
  Data Store Read1/1 -> Product1/1

== system CF009A_GmOvrlStMgr/GmOvrlStMgr/GmOvrlStMgrPer1/LKAIntv/HwTqLkaTqSignNotEqu/ChkTmr1/GetTiSpan100MicroSec32bit ==
  note: Subtract original reference time
  note: seconds
  note: microseconds
  note: counts
  note: Wrap-to-zero
  note: 1 count = 100 uSec
  note: Get current system time
  note: GetTiSpan100MicroSec32bit
  note: Created Aug 18, 2015
      | Modified Oct 21, 2015
      | Modified Oct 30, 2015
      | Kevin Derry
  RefTmr : Inport
  CopyRight2 : Subsystem  Description=|  mask(Copyright Information){none=on}
      | Copyright info block.                                               
      |                                                                     
      | Place copyright information at the top of every subsystem in design.
      mask prompts: none "No parameters"
      mask help: Place copyright information at the top of every subsystem in design.
      mask Display:
      | NxtrConf = 'Nexteer Confidential';
      | 
      | sys = bdroot; %handle for the current model ("system")
      | first = get_param(sys,'Created');
      | if(isempty(first))
      |     first = datestr(now,'yyyy');
      | else
      |     first = first(end-3:end);  %year is last four digits
      | end
      | 
      | last = get_param(sys,'LastModifiedDate');
      | if isempty(last)
      |     last = datestr(now,'yyyy');
      | else
      |     last = last(end-3:end);
      | end
      | 
      | if strcmp(first,last)
      |     fprintf('%s -- Copyright %s Nexteer',NxtrConf,first)
      | else
      |     fprintf('%s -- %s%s- %s Nexteer',NxtrConf,char(169),first,last)
      | end
  Count per uSec : Constant  Value=0.01
  Data Store Read1 : DataStoreRead  DataStoreName=SimnTi
  Data Type Conversion2 : DataTypeConversion  OutDataTypeStr=uint32
  Divide1 : Product  Inputs=**
  Divide2 : Product  Inputs=*/
  If : If  NumInputs=2  IfExpression=u1 >= u2
  Max Counts : Constant  Value=2^32-1
  Merge : Merge
  No wrapping : Subsystem  TreatAsAtomicUnit=on
  Product2 : Product
  Product3 : Product
  Rounding : Rounding
  Subtract3 : Sum  Inputs=+-
  Wrapping : Subsystem  TreatAsAtomicUnit=on
  uSec per Sec : Constant  Value=1000000
  TiSpan : Outport
  wires:
  Wrapping/1(Out1) -> Merge/2
  No wrapping/1(Out1) -> Merge/1
  If/2 -> Wrapping/Action
  If/1 -> No wrapping/Action
  Product3/1 -> Subtract3/2
  Subtract3/1 -> Data Type Conversion2/1
  Rounding/1 -> Product3/1
  Divide2/1 -> Rounding/1
  Max Counts/1 -> Divide2/2, Product3/2
  Divide1/1 -> Divide2/1, Subtract3/1
  Product2/1 -> Divide1/1
  Data Store Read1/1 -> Product2/1
  Count per uSec/1 -> Divide1/2
  uSec per Sec/1 -> Product2/2
  Merge/1 -> TiSpan/1
  RefTmr/1 -> If/2, No wrapping/2(ref), Wrapping/2(ref)
  Data Type Conversion2/1 -> If/1, No wrapping/1(new), Wrapping/1(new)

== system CF009A_GmOvrlStMgr/GmOvrlStMgr/GmOvrlStMgrPer1/LKAIntv/HwTqLkaTqSignNotEqu/ChkTmr1/LKAIntvTi1Elpd ==
  Action Port : ActionPort  ActionType=then
  Constant13 : Constant  RequirementInfo={} %GIDa_b4f81cfb_baa7_47ff_8045_f18810ae4b25  Value=true  OutDataTypeStr=boolean
      settings: AttributesFormatString=%<OutDataTypeStr>
  CopyRight2 : Subsystem  Description=|  mask(Copyright Information){none=on}
      | Copyright info block.                                               
      |                                                                     
      | Place copyright information at the top of every subsystem in design.
      mask prompts: none "No parameters"
      mask help: Place copyright information at the top of every subsystem in design.
      mask Display:
      | NxtrConf = 'Nexteer Confidential';
      | 
      | sys = bdroot; %handle for the current model ("system")
      | first = get_param(sys,'Created');
      | if(isempty(first))
      |     first = datestr(now,'yyyy');
      | else
      |     first = first(end-3:end);  %year is last four digits
      | end
      | 
      | last = get_param(sys,'LastModifiedDate');
      | if isempty(last)
      |     last = datestr(now,'yyyy');
      | else
      |     last = last(end-3:end);
      | end
      | 
      | if strcmp(first,last)
      |     fprintf('%s -- Copyright %s Nexteer',NxtrConf,first)
      | else
      |     fprintf('%s -- %s%s- %s Nexteer',NxtrConf,char(169),first,last)
      | end
  Out1 : Outport
  wires:
  Constant13/1 -> Out1/1

== system CF009A_GmOvrlStMgr/GmOvrlStMgr/GmOvrlStMgrPer1/LKAIntv/HwTqLkaTqSignNotEqu/ChkTmr1/LKAIntvTi1NotElpd ==
  Action Port : ActionPort  ActionType=else
  CopyRight2 : Subsystem  Description=|  mask(Copyright Information){none=on}
      | Copyright info block.                                               
      |                                                                     
      | Place copyright information at the top of every subsystem in design.
      mask prompts: none "No parameters"
      mask help: Place copyright information at the top of every subsystem in design.
      mask Display:
      | NxtrConf = 'Nexteer Confidential';
      | 
      | sys = bdroot; %handle for the current model ("system")
      | first = get_param(sys,'Created');
      | if(isempty(first))
      |     first = datestr(now,'yyyy');
      | else
      |     first = first(end-3:end);  %year is last four digits
      | end
      | 
      | last = get_param(sys,'LastModifiedDate');
      | if isempty(last)
      |     last = datestr(now,'yyyy');
      | else
      |     last = last(end-3:end);
      | end
      | 
      | if strcmp(first,last)
      |     fprintf('%s -- Copyright %s Nexteer',NxtrConf,first)
      | else
      |     fprintf('%s -- %s%s- %s Nexteer',NxtrConf,char(169),first,last)
      | end
  Data Store Read : DataStoreRead  DataStoreName=LkaIntvPrev
  Out1 : Outport
  wires:
  Data Store Read/1 -> Out1/1

== system CF009A_GmOvrlStMgr/GmOvrlStMgr/GmOvrlStMgrPer1/LKAIntv/HwTqLkaTqSignNotEqu/ChkTmr2/CopyRight2 ==

== system CF009A_GmOvrlStMgr/GmOvrlStMgr/GmOvrlStMgrPer1/LKAIntv/HwTqLkaTqSignNotEqu/ChkTmr2/GetRefTmr100MicroSec32bit ==
  note: Created Aug 18, 2015
      | Modified Oct 21, 2015
      | Modified Oct 30, 2015
      | Kevin Derry
  note: GetRefTmr100MicroSec32bit
  note: Wrap-to-zero
  note: counts
  note: microseconds
  note: seconds
  note: 1 count = 100 uSec
  CopyRight2 : Subsystem  Description=|  mask(Copyright Information){none=on}
      | Copyright info block.                                               
      |                                                                     
      | Place copyright information at the top of every subsystem in design.
      mask prompts: none "No parameters"
      mask help: Place copyright information at the top of every subsystem in design.
      mask Display:
      | NxtrConf = 'Nexteer Confidential';
      | 
      | sys = bdroot; %handle for the current model ("system")
      | first = get_param(sys,'Created');
      | if(isempty(first))
      |     first = datestr(now,'yyyy');
      | else
      |     first = first(end-3:end);  %year is last four digits
      | end
      | 
      | last = get_param(sys,'LastModifiedDate');
      | if isempty(last)
      |     last = datestr(now,'yyyy');
      | else
      |     last = last(end-3:end);
      | end
      | 
      | if strcmp(first,last)
      |     fprintf('%s -- Copyright %s Nexteer',NxtrConf,first)
      | else
      |     fprintf('%s -- %s%s- %s Nexteer',NxtrConf,char(169),first,last)
      | end
  Count per uSec : Constant  Value=0.01
  Data Store Read1 : DataStoreRead  DataStoreName=SimnTi
  Data Type Conversion1 : DataTypeConversion  OutDataTypeStr=uint32
  Divide1 : Product  Inputs=**
  Divide2 : Product  Inputs=*/
  Max Counts : Constant  Value=2^32-1
  Product1 : Product
  Product2 : Product
  Rounding : Rounding
  Subtract1 : Sum  Inputs=+-
  uSec per Sec : Constant  Value=1000000
  RefTmr : Outport
  wires:
  Data Store Read1/1 -> Product1/1
  Data Type Conversion1/1 -> RefTmr/1
  uSec per Sec/1 -> Product1/2
  Count per uSec/1 -> Divide1/2
  Product1/1 -> Divide1/1
  Divide1/1 -> Subtract1/1, Divide2/1
  Max Counts/1 -> Product2/2, Divide2/2
  Divide2/1 -> Rounding/1
  Rounding/1 -> Product2/1
  Subtract1/1 -> Data Type Conversion1/1
  Product2/1 -> Subtract1/2
